simulink model "system_model"  (R2022b)
settings: Solver=FixedStepAuto  StartTime=0.0  StopTime=10  RelTol=1e-3
values from neighbouring files (symbols this model uses):
  init_theta_1 = pi    (= 3.14159265359)    [Copy_of_step2_whitebox_beam.m]    (also in compare_ourmodel_with_others.m = 0; linearize_script.m; step2_whitebox_beam.m; syms_test.m)
  init_theta_2 = -pi/2    (= -1.57079632679)    [Copy_of_step2_whitebox_beam.m]    (also in compare_ourmodel_with_others.m = 0; linearize_script.m = 1.57079632679; step2_whitebox_beam.m; syms_test.m = 0)
settings Model: Creator=97083  LastModifiedBy=97083
settings DataIOCC: ExternalInput=[u]
settings DebuggingCC: UnderSpecifiedDimensionMsg=warning

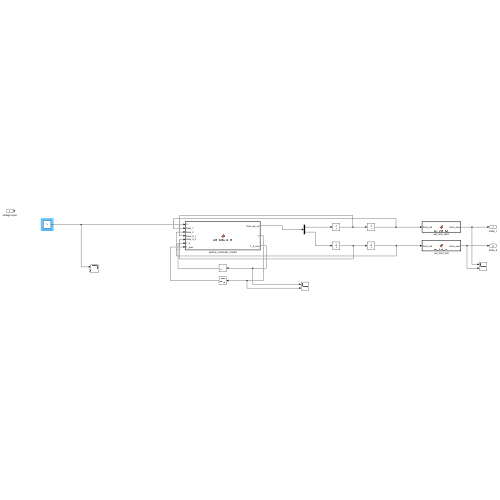
[thumbnail: Simulink's stored preview of the top-level diagram]
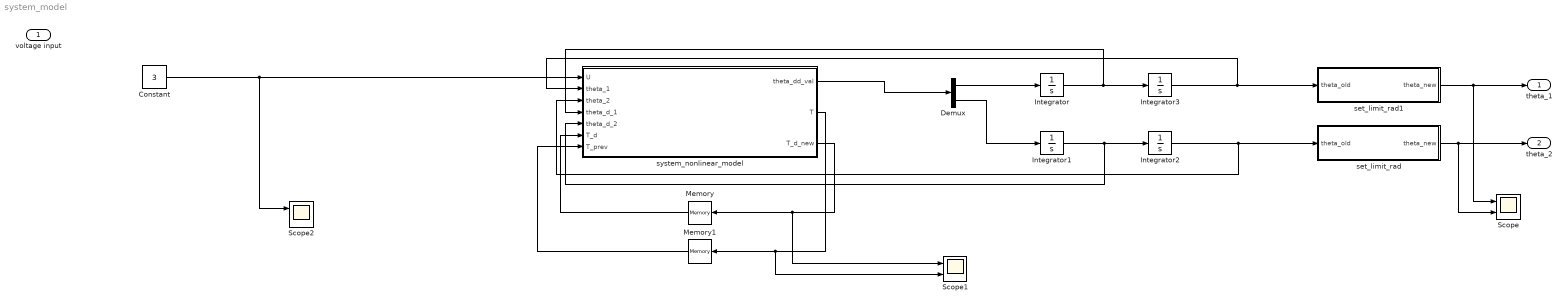
== system system_model ==
  voltage input : Inport  LockScale=on
  Constant : Constant  Value=3
  Demux : Demux  Outputs=2
  Integrator : Integrator
  Integrator1 : Integrator
  Integrator2 : Integrator  InitialCondition=init_theta_2
  Integrator3 : Integrator  InitialCondition=init_theta_1
  Memory : Memory  InheritSampleTime=on
  Memory1 : Memory  InheritSampleTime=on
  Scope : Scope  NumInputPorts=2
  Scope1 : Scope  NumInputPorts=2
  Scope2 : Scope  NumInputPorts=2
  set_limit_rad : MATLAB Function  TreatAsAtomicUnit=on
  set_limit_rad1 : MATLAB Function  TreatAsAtomicUnit=on
  system_nonlinear_model : MATLAB Function  TreatAsAtomicUnit=on
  theta_1 : Outport
  theta_2 : Outport  Port=2
  wires:
  system_nonlinear_model/1(theta_dd_val) -> Demux/1
  Demux/1 -> Integrator/1
  Integrator/1 -> system_nonlinear_model/4(theta_d_1), Integrator3/1
  Demux/2 -> Integrator1/1
  Integrator1/1 -> system_nonlinear_model/5(theta_d_2), Integrator2/1
  Integrator3/1 -> set_limit_rad1/1(theta_old), system_nonlinear_model/2(theta_1)
  Integrator2/1 -> system_nonlinear_model/3(theta_2), set_limit_rad/1(theta_old)
  set_limit_rad/1(theta_new) -> Scope/2, theta_2/1
  set_limit_rad1/1(theta_new) -> Scope/1, theta_1/1
  Constant/1 -> Scope2/1, system_nonlinear_model/1(U)
  system_nonlinear_model/3(T_d_new) -> Scope1/1, Memory/1
  Memory/1 -> system_nonlinear_model/6(T_d)
  system_nonlinear_model/2(T) -> Scope1/2, Memory1/1
  Memory1/1 -> system_nonlinear_model/7(T_prev)

== matlab function system_model/set_limit_rad ==
  settings: updateMethod=DISCRETE  sampleTime=0.001
  data: theta_old input size=1; theta_new output size=1
function theta_new   = set_limit_rad(theta_old)

theta_new = theta_old - floor(theta_old / 2 / pi) * 2 * pi;
theta_new = theta_old;

== matlab function system_model/system_nonlinear_model ==
  settings: updateMethod=DISCRETE  sampleTime=0.001
  data: U input size=1; theta_dd_val output size=2; T output; theta_1 input size=1; theta_2 input size=1; theta_d_1 input size=1; theta_d_2 input size=1; T_d input; T_prev input; T_d_new output
function [theta_dd_val, T, T_d_new]   = get_theta_dt_dt(U, theta_1, theta_2, theta_d_1, theta_d_2, T_d, T_prev)


u = U(1);
k_m_0 = 15;
tau_e_0 = 0.03;

T = k_m_0 * u - tau_e_0 * T_d;



theta_dd_val = [
                                                                                                       (50632000000*((3*T_d)/100 - 15*u))/(7*(3388000*cos(theta_2)^2 - 1450246047)) - theta_d_2*((160*(7700*cos(theta_2) + 6329))/(7*(3388000*cos(theta_2)^2 - 1450246047)) + (50632000000*sin(theta_2)*((77*theta_d_1)/200000 + (77*theta_d_2)/200000))/(7*(3388000*cos(theta_2)^2 - 1450246047))) - (50632000000*((75537*sin(theta_1 + theta_2))/2000000 + (38259*sin(theta_1))/800000))/(7*(3388000*cos(theta_2)^2 - 1450246047)) - theta_d_1*((50632000000*((77*theta_d_2*sin(theta_2))/200000 - 5171/250))/(7*(3388000*cos(theta_2)^2 - 1450246047)) + (440*theta_d_1*sin(theta_2)*(7700*cos(theta_2) + 6329))/(3388000*cos(theta_2)^2 - 1450246047)) + (43164*sin(theta_1 + theta_2)*(7700*cos(theta_2) + 6329))/(3388000*cos(theta_2)^2 - 1450246047);
theta_d_2*((80*(30800*cos(theta_2) + 8032663))/(7*(3388000*cos(theta_2)^2 - 1450246047)) + (8000000*sin(theta_2)*((77*theta_d_1)/200000 + (77*theta_d_2)/200000)*(7700*cos(theta_2) + 6329))/(7*(3388000*cos(theta_2)^2 - 1450246047))) + theta_d_1*((8000000*((77*theta_d_2*sin(theta_2))/200000 - 5171/250)*(7700*cos(theta_2) + 6329))/(7*(3388000*cos(theta_2)^2 - 1450246047)) + (220*theta_d_1*sin(theta_2)*(30800*cos(theta_2) + 8032663))/(3388000*cos(theta_2)^2 - 1450246047)) - (21582*sin(theta_1 + theta_2)*(30800*cos(theta_2) + 8032663))/(3388000*cos(theta_2)^2 - 1450246047) + (8000000*(7700*cos(theta_2) + 6329)*((75537*sin(theta_1 + theta_2))/2000000 + (38259*sin(theta_1))/800000))/(7*(3388000*cos(theta_2)^2 - 1450246047)) - (8000000*(7700*cos(theta_2) + 6329)*((3*T_d)/100 - 15*u))/(7*(3388000*cos(theta_2)^2 - 1450246047))];
 
%                                                                                                         (43164*sin(theta_1 + theta_2)*(7700*cos(theta_2) + 6329))/(3388000*cos(theta_2)^2 - 1450246047) - (759480000000*u)/(7*(3388000*cos(theta_2)^2 - 1450246047)) - theta_d_2*((160*(7700*cos(theta_2) + 6329))/(7*(3388000*cos(theta_2)^2 - 1450246047)) + (50632000000*sin(theta_2)*((77*theta_d_1)/200000 + (77*theta_d_2)/200000))/(7*(3388000*cos(theta_2)^2 - 1450246047))) - (50632000000*((75537*sin(theta_1 + theta_2))/2000000 + (38259*sin(theta_1))/800000))/(7*(3388000*cos(theta_2)^2 - 1450246047)) - theta_d_1*((50632000000*((77*theta_d_2*sin(theta_2))/200000 - 5171/250))/(7*(3388000*cos(theta_2)^2 - 1450246047)) + (440*theta_d_1*sin(theta_2)*(7700*cos(theta_2) + 6329))/(3388000*cos(theta_2)^2 - 1450246047))
% theta_d_2*((80*(30800*cos(theta_2) + 8032663))/(7*(3388000*cos(theta_2)^2 - 1450246047)) + (8000000*sin(theta_2)*((77*theta_d_1)/200000 + (77*theta_d_2)/200000)*(7700*cos(theta_2) + 6329))/(7*(3388000*cos(theta_2)^2 - 1450246047))) + theta_d_1*((8000000*((77*theta_d_2*sin(theta_2))/200000 - 5171/250)*(7700*cos(theta_2) + 6329))/(7*(3388000*cos(theta_2)^2 - 1450246047)) + (220*theta_d_1*sin(theta_2)*(30800*cos(theta_2) + 8032663))/(3388000*cos(theta_2)^2 - 1450246047)) + (120000000*u*(7700*cos(theta_2) + 6329))/(7*(3388000*cos(theta_2)^2 - 1450246047)) - (21582*sin(theta_1 + theta_2)*(30800*cos(theta_2) + 8032663))/(3388000*cos(theta_2)^2 - 1450246047) + (8000000*(7700*cos(theta_2) + 6329)*((75537*sin(theta_1 + theta_2))/2000000 + (38259*sin(theta_1))/800000))/(7*(3388000*cos(theta_2)^2 - 1450246047))
%  

T_d_new = (T - T_prev)/1;

== matlab function system_model/set_limit_rad1 ==
  settings: updateMethod=DISCRETE  sampleTime=0.001
  data: theta_old input size=1; theta_new output size=1
function theta_new   = set_limit_rad(theta_old)

theta_new = theta_old - floor(theta_old / 2 / pi) * 2 * pi;
theta_new = theta_old;
